simulink model "sine_wave"  (R2021b)
settings: Solver=VariableStepAuto  StartTime=0.0  StopTime=10.0  RelTol=1e-3
settings Model: Creator=DELL  LastModifiedBy=DELL

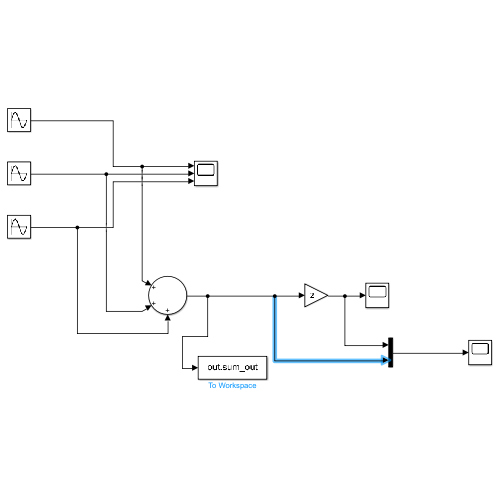
[thumbnail: Simulink's stored preview of the top-level diagram]
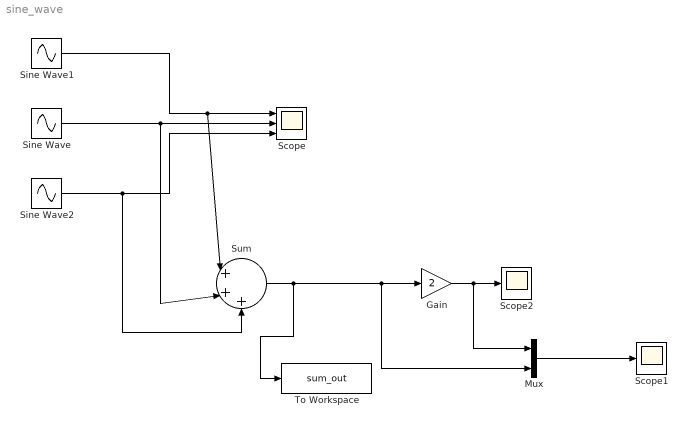
== system sine_wave ==
  Gain : Gain  Gain=2
  Mux : Mux  Inputs=2
  Scope : Scope  NumInputPorts=3
  Scope1 : Scope
  Scope2 : Scope
  Sine Wave : Sin  Frequency=5  SampleTime=0
  Sine Wave1 : Sin  SampleTime=0
  Sine Wave2 : Sin  Frequency=3  SampleTime=0
  Sum : Sum  Inputs=|+++
  To Workspace : ToWorkspace  VariableName=sum_out  SaveFormat=Timeseries  SampleTime=-1
  wires:
  Sine Wave1/1 -> Sum/1, Scope/1
  Sine Wave/1 -> Sum/2, Scope/2
  Sine Wave2/1 -> Sum/3, Scope/3
  Gain/1 -> Mux/1, Scope2/1
  Sum/1 -> To Workspace/1, Mux/2, Gain/1
  Mux/1 -> Scope1/1
